simulink model "eq6_6__6_9"  (R2020a)
settings: Solver=VariableStepAuto  StartTime=0.0  StopTime=10.0  RelTol=1e-3
settings Model: Creator=shrad  LastModifiedBy=shrad

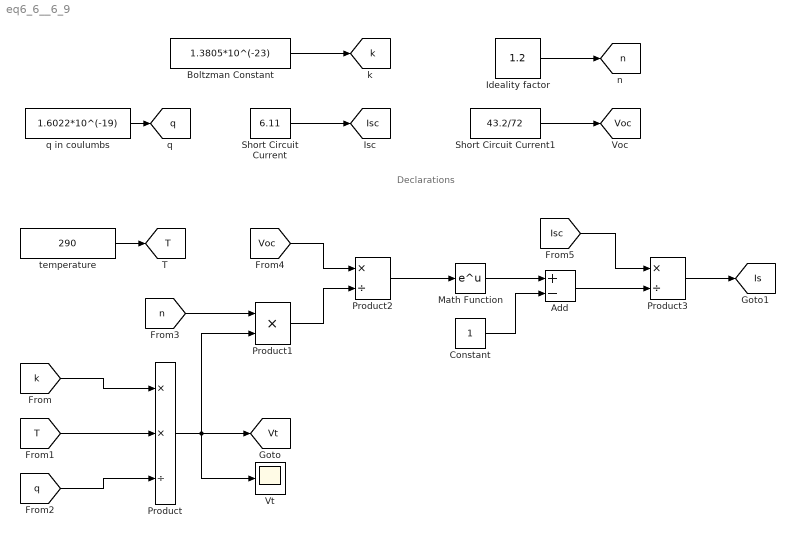
== system eq6_6__6_9 ==
  note: Declarations
  Add : Sum  Inputs=+-
  Boltzman Constant : Constant  Value=1.3805*10^(-23)
  Constant : Constant
  Ideality factor : Constant  Value=1.2
  Math Function : Math  SaturateOnIntegerOverflow=on
  Product : Product  Inputs=**/
  Product1 : Product
  Product2 : Product  Inputs=*/
  Product3 : Product  Inputs=*/
  Short Circuit Current : Constant  Value=6.11
  Short Circuit Current1 : Constant  Value=43.2/72
  Vt : Scope
  q in coulumbs : Constant  Value=1.6022*10^(-19)
  temperature : Constant  Value=290
  tag scope: Is=global, Isc=global, T=global, Voc=global, Vt=global, k=global, n=global, q=global
  wires:
  Product2/1 -> Math Function/1
  Product/1 -> Product1/2, Vt/1, [Vt]
  [Isc] -> Product3/1
  [n] -> Product1/1
  Add/1 -> Product3/2
  Product1/1 -> Product2/2
  [Voc] -> Product2/1
  Constant/1 -> Add/2
  [T] -> Product/2
  [q] -> Product/3
  [k] -> Product/1
  Product3/1 -> [Is]
  Math Function/1 -> Add/1
  Short Circuit Current1/1 -> [Voc]
  Ideality factor/1 -> [n]
  Boltzman Constant/1 -> [k]
  Short Circuit Current/1 -> [Isc]
  q in coulumbs/1 -> [q]
  temperature/1 -> [T]
